simulink model "product_collapse_test_3"  (R2015a)
settings: Solver=ode45  StartTime=0.0  StopTime=10.0  RelTol=1e-3
model workspace (MAT data in the model file):
  Var = 0
  Var1 = 0
  lustrec_slx_eps = 0.5
settings Model: Creator=arnaud  LastModifiedBy=hbourbou
settings DataIOCC: SaveFormat=Structure  SignalLoggingSaveFormat=ModelDataLogs
settings OptimizationCC: ExpressionDepthLimit=2147483647
settings DebuggingCC: UnderspecifiedInitializationDetection=Classic  MergeDetectMultiDrivingBlocksExec=none  SolverPrmCheckMsg=warning  FcnCallInpInsideContextMsg=EnableAllAsWarning  StateNameClashWarn=warning  StrictBusMsg=Warning
settings GRTTargetCC: CombineOutputUpdateFcns=off  GRTInterface=on

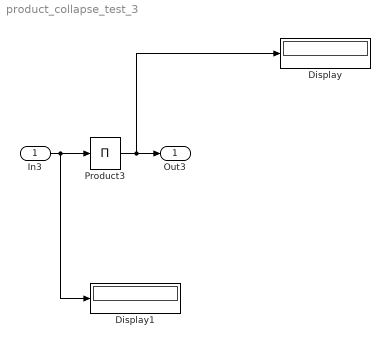
== system product_collapse_test_3 ==
  In3 : Inport  OutMin=-10.  OutMax=10.  PortDimensions=[2 3]
  Display : Display
  Display1 : Display
  Product3 : Product  Inputs=1  RndMeth=Zero
  Out3 : Outport
  wires:
  In3/1 -> Display1/1, Product3/1
  Product3/1 -> Display/1, Out3/1
